simulink model "SimulinkComunicacionVuelta"  (R2015b)
settings: Solver=FixedStepAuto  StartTime=0.0  StopTime=inf  FixedStep=0.1  RelTol=1e-3
undefined symbols (not defined in the file or in its folder): serial
libraries: instrumentlib x3
settings Model: Creator=nico  LastModifiedBy=nico
settings DataIOCC: SaveFormat=Array
settings DebuggingCC: UnderspecifiedInitializationDetection=Classic  MergeDetectMultiDrivingBlocksExec=none  SolverPrmCheckMsg=warning
settings HardwareCC: ProdBitPerPointer=32  ProdLargestAtomicFloat=None  ProdIntDivRoundTo=Undefined  ProdEndianess=Unspecified  ProdWordSize=32  ProdHWDeviceType=32-bit Generic
settings GRTTargetCC: GeneratePreprocessorConditionals=Disable all
settings ConfigComp: CovModelRefEnable=Off

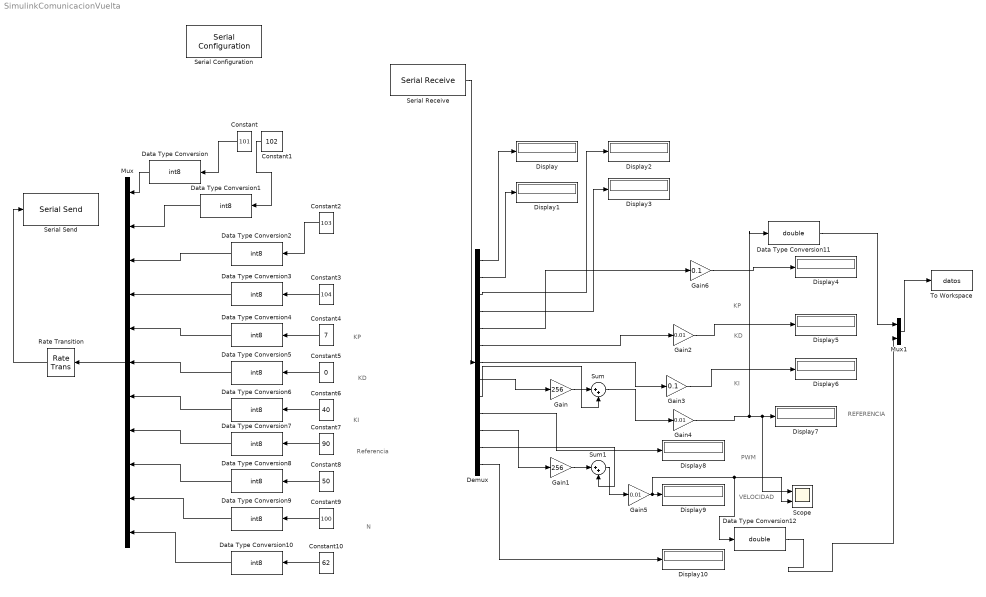
== system SimulinkComunicacionVuelta ==
  note: N
  note: Referencia
  note: KI
  note: KD
  note: KP
  note: VELOCIDAD
  note: PWM
  note: REFERENCIA
  note: KI
  note: KD
  note: KP
  Constant : Constant  Value=101  SampleTime=0.5
  Constant1 : Constant  Value=102  SampleTime=0.5
  Constant10 : Constant  Value=62  SampleTime=0.5
  Constant2 : Constant  Value=103  SampleTime=0.5
  Constant3 : Constant  Value=104  SampleTime=0.5
  Constant4 : Constant  Value=7  SampleTime=0.5
  Constant5 : Constant  Value=0  SampleTime=0.5
  Constant6 : Constant  Value=40  SampleTime=0.5
  Constant7 : Constant  Value=90  SampleTime=0.5
  Constant8 : Constant  Value=50  SampleTime=0.5
  Constant9 : Constant  Value=100  SampleTime=0.5
  Data Type Conversion{,1..10} (11 alike) : DataTypeConversion  OutDataTypeStr=int8
  Data Type Conversion11 : DataTypeConversion  OutDataTypeStr=double
  Data Type Conversion12 : DataTypeConversion  OutDataTypeStr=double
  Demux : Demux  Outputs=13
  Display{,1..10} (11 alike) : Display
      Display7 settings: Decimation=3
  Gain : Gain  Gain=256
  Gain1 : Gain  Gain=256
  Gain2 : Gain  Gain=0.01
  Gain3 : Gain  Gain=0.1
  Gain4 : Gain  Gain=0.01
  Gain5 : Gain  Gain=0.01
  Gain6 : Gain  Gain=0.1
  Mux : Mux  Inputs=11
  Mux1 : Mux  Inputs=2
  Rate Transition : RateTransition  OutPortSampleTimeOpt=Multiple of input port sample time
  Scope : Scope  NumInputPorts=2
  Serial Configuration : instrumentlib/Serial Configuration  Priority=-200000  ComPortMenu=<Please select a port...>  ComPort=COM3  ObjConstructor=serial('COM3');  BaudRate=9600  DataBits=8  Parity=none  StopBits=1  FlowControl=none  Timeout=20  ByteOrder=LittleEndian
  Serial Receive : instrumentlib/Serial Receive  ComPortMenu=<Please select a port...>  ComPort=COM3  ObjConstructor=serial('COM3');  Terminator=<none>  DataSize="[13   1]"  DataType=uint8  EnableBlockingMode=on  ActionDataUnavailable=Output last received value  CustomValue=0  SampleTime=0.2
  Serial Send : instrumentlib/Serial Send  ComPortMenu=<Please select a port...>  ComPort=COM3  ObjConstructor=serial('COM3');  Terminator=<none>  EnableBlockingMode=on
  Sum : Sum  Inputs=|++
  Sum1 : Sum  Inputs=|++
  To Workspace : ToWorkspace  VariableName=datos  SaveFormat=Timeseries  SampleTime=-1
  wires:
  Constant/1 -> Data Type Conversion/1
  Data Type Conversion/1 -> Mux/1
  Serial Receive/1 -> Demux/1
  Demux/1 -> Display/1
  Constant1/1 -> Data Type Conversion1/1
  Data Type Conversion1/1 -> Mux/2
  Demux/2 -> Display1/1
  Mux/1 -> Rate Transition/1
  Demux/4 -> Display3/1
  Demux/3 -> Display2/1
  Gain/1 -> Sum/1
  Demux/8 -> Gain/1
  Demux/9 -> Sum/2
  Demux/10 -> Display8/1
  Demux/11 -> Gain1/1
  Demux/12 -> Sum1/2
  Gain1/1 -> Sum1/1
  Data Type Conversion2/1 -> Mux/3
  Constant2/1 -> Data Type Conversion2/1
  Data Type Conversion3/1 -> Mux/4
  Constant3/1 -> Data Type Conversion3/1
  Data Type Conversion4/1 -> Mux/5
  Constant4/1 -> Data Type Conversion4/1
  Data Type Conversion5/1 -> Mux/6
  Constant5/1 -> Data Type Conversion5/1
  Data Type Conversion6/1 -> Mux/7
  Constant6/1 -> Data Type Conversion6/1
  Data Type Conversion7/1 -> Mux/8
  Constant7/1 -> Data Type Conversion7/1
  Data Type Conversion9/1 -> Mux/10
  Data Type Conversion8/1 -> Mux/9
  Constant8/1 -> Data Type Conversion8/1
  Constant9/1 -> Data Type Conversion9/1
  Gain2/1 -> Display5/1
  Demux/6 -> Gain2/1
  Gain3/1 -> Display6/1
  Demux/7 -> Gain3/1
  Sum/1 -> Gain4/1
  Gain5/1 -> Data Type Conversion12/1, Scope/2, Display9/1
  Sum1/1 -> Gain5/1
  Gain4/1 -> Data Type Conversion11/1, Scope/1, Display7/1
  Rate Transition/1 -> Serial Send/1
  Constant10/1 -> Data Type Conversion10/1
  Data Type Conversion10/1 -> Mux/11
  Gain6/1 -> Display4/1
  Demux/5 -> Gain6/1
  Demux/13 -> Display10/1
  Data Type Conversion12/1 -> Mux1/2
  Mux1/1 -> To Workspace/1
  Data Type Conversion11/1 -> Mux1/1
